simulink model "Problem3_sim"  (R2018a)
settings: Solver=ode45  StartTime=0.0  StopTime=sim_time  RelTol=1e-3
values from neighbouring files (symbols this model uses):
  g = 9.81    [Problem3.m]
  kd_fi = (2*zeta_fi*omega_fi-alpha_fi1)/alpha_fi2    [Problem3.m]
  ki_chi = omega_chi^2*V_g/g    [Problem3.m]
  ki_fi = -0    (= 0)    [Problem3.m]
  kp_chi = 2*zeta_chi*omega_chi*V_g/g    [Problem3.m]
  kp_fi = -2    [Problem3.m]
  sim_time = 600    [Problem3.m]
  V_g = 580/3.6    (= 161.111111111)    [Problem3.m]
undefined symbols (not defined in the file or in its folder): data
libraries: simulink_extras x2
settings Model: Creator=marti  LastModifiedBy=Anders Vagle
settings OptimizationCC: LifeSpan=inf
settings DebuggingCC: SFExecutionAtInitializationDiag=none
settings HardwareCC: ProdBitPerSizeT=32  ProdBitPerPtrDiffT=32  ProdWordSize=32  ProdHWDeviceType=Specified
settings CodeAppCC: StateflowObjectComments=on

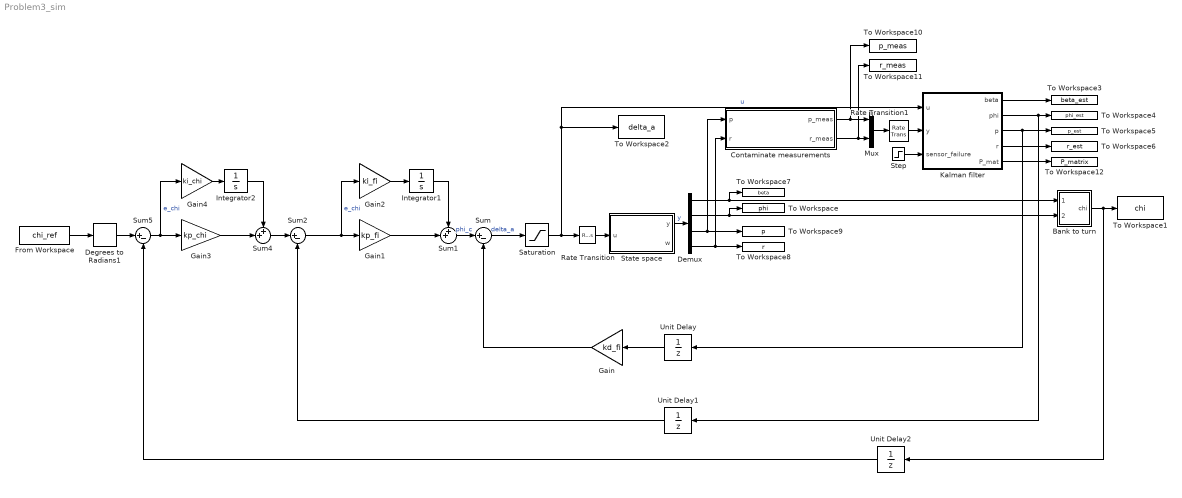
== system Problem3_sim ==
  Bank to turn : Subsystem
  Contaminate measurements : MATLAB Function  TreatAsAtomicUnit=on
  Degrees to Radians1 : simulink_extras/Transformations/Degrees to Radians
  Demux : Demux
  From Workspace : FromWorkspace  VariableName=chi_ref  SampleTime=0  Interpolate=off  OutputAfterFinalValue=Holding final value
  Gain : Gain  Gain=kd_fi
  Gain1 : Gain  Gain=kp_fi
  Gain2 : Gain  Gain=ki_fi
  Gain3 : Gain  Gain=kp_chi
  Gain4 : Gain  Gain=ki_chi
  Integrator1 : Integrator
  Integrator2 : Integrator
  Kalman filter : MATLAB Function  TreatAsAtomicUnit=on  mask{data=data}
      mask prompts: data "data struct"
  Mux : Mux  Inputs=2
  Rate Transition : RateTransition  OutPortSampleTime=Ts
  Rate Transition1 : RateTransition
  Saturation : Saturate  UpperLimit=30/180*pi  LowerLimit=-30/180*pi
  State space : MATLAB Function  TreatAsAtomicUnit=on
  Step : Step  Time=sim_time*2  SampleTime=0
  Sum : Sum  Inputs=|+-
  Sum1 : Sum  Inputs=++|
  Sum2 : Sum  Inputs=|+-
  Sum4 : Sum  Inputs=++|
  Sum5 : Sum  Inputs=|+-
  To Workspace : ToWorkspace  VariableName=phi  SaveFormat=Timeseries  SampleTime=-1
  To Workspace1 : ToWorkspace  VariableName=chi  SaveFormat=Timeseries  SampleTime=-1
  To Workspace10 : ToWorkspace  VariableName=p_meas  SaveFormat=Timeseries  SampleTime=-1
  To Workspace11 : ToWorkspace  VariableName=r_meas  SaveFormat=Timeseries  SampleTime=-1
  To Workspace12 : ToWorkspace  VariableName=P_matrix  SampleTime=-1
  To Workspace2 : ToWorkspace  VariableName=delta_a  SaveFormat=Timeseries  SampleTime=-1
  To Workspace3 : ToWorkspace  VariableName=beta_est  SaveFormat=Timeseries  SampleTime=-1
  To Workspace4 : ToWorkspace  VariableName=phi_est  SaveFormat=Timeseries  SampleTime=-1
  To Workspace5 : ToWorkspace  VariableName=p_est  SaveFormat=Timeseries  SampleTime=-1
  To Workspace6 : ToWorkspace  VariableName=r_est  SaveFormat=Timeseries  SampleTime=-1
  To Workspace7 : ToWorkspace  VariableName=beta  SaveFormat=Timeseries  SampleTime=-1
  To Workspace8 : ToWorkspace  VariableName=r  SaveFormat=Timeseries  SampleTime=-1
  To Workspace9 : ToWorkspace  VariableName=p  SaveFormat=Timeseries  SampleTime=-1
  Unit Delay : UnitDelay  SampleTime=-1
  Unit Delay1 : UnitDelay  SampleTime=-1
  Unit Delay2 : UnitDelay  SampleTime=-1
  wires:
  Gain/1 -> Sum/2
  Sum1/1 -> Sum/1  "phi_c"
  Integrator1/1 -> Sum1/1
  Gain1/1 -> Sum1/2
  Sum2/1 -> Gain2/1, Gain1/1  "e_chi"
  Demux/2 -> To Workspace/1, Bank to turn/2(phi)
  Integrator2/1 -> Sum4/1
  Gain3/1 -> Sum4/2
  Sum5/1 -> Gain4/1, Gain3/1  "e_chi"
  Sum/1 -> Saturation/1  "delta_a"
  Sum4/1 -> Sum2/1
  Degrees to Radians1/1 -> Sum5/1
  From Workspace/1 -> Degrees to Radians1/1
  Demux/1 -> To Workspace7/1, Bank to turn/1(beta)
  Saturation/1 -> Rate Transition/1, Kalman filter/1(u), To Workspace2/1  "u"
  State space/1(y) -> Demux/1  "y"
  Demux/3 -> To Workspace9/1, Contaminate measurements/1(p)
  Gain2/1 -> Integrator1/1
  Gain4/1 -> Integrator2/1
  Demux/4 -> Contaminate measurements/2(r), To Workspace8/1
  Contaminate measurements/2(r_meas) -> To Workspace11/1, Mux/2
  Contaminate measurements/1(p_meas) -> Mux/1, To Workspace10/1
  Kalman filter/1(beta) -> To Workspace3/1
  Kalman filter/2(phi) -> Unit Delay1/1, To Workspace4/1
  Kalman filter/3(p) -> Unit Delay/1, To Workspace5/1
  Kalman filter/4(r) -> To Workspace6/1
  Rate Transition/1 -> State space/1(u)
  Unit Delay/1 -> Gain/1
  Unit Delay1/1 -> Sum2/2
  Mux/1 -> Rate Transition1/1
  Rate Transition1/1 -> Kalman filter/2(y)
  Unit Delay2/1 -> Sum5/2
  Bank to turn/1(chi) -> To Workspace1/1, Unit Delay2/1
  Kalman filter/5(P_mat) -> To Workspace12/1
  Step/1 -> Kalman filter/3(sensor_failure)

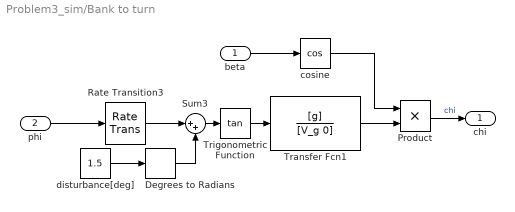
== system Problem3_sim/Bank to turn ==
  beta : Inport
  phi : Inport  Port=2
  Degrees to Radians : simulink_extras/Transformations/Degrees to Radians
  Product : Product
  Rate Transition3 : RateTransition  OutPortSampleTime=Ts
  Sum3 : Sum  Inputs=|++
  Transfer Fcn1 : TransferFcn  Numerator=[g]  Denominator=[V_g 0]
  Trigonometric Function : Trigonometry  Operator=tan
  cosine : Trigonometry  Operator=cos
  disturbance[deg] : Constant  Value=1.5
  chi : Outport
  wires:
  cosine/1 -> Product/1
  phi/1 -> Rate Transition3/1
  beta/1 -> cosine/1
  disturbance[deg]/1 -> Degrees to Radians/1
  Trigonometric Function/1 -> Transfer Fcn1/1
  Rate Transition3/1 -> Sum3/1
  Sum3/1 -> Trigonometric Function/1
  Degrees to Radians/1 -> Sum3/2
  Transfer Fcn1/1 -> Product/2
  Product/1 -> chi/1  "chi"

== matlab function Problem3_sim/Contaminate measurements ==
  data: p input; p_meas output; r input; r_meas output
function [p_meas, r_meas] = contaminate(p, r)

% persistent counter; % Variable for checking if it is the first iteration.
% coder.extrinsic('randn','rng');
% if isempty(counter)
%    counter = 1;
%    rng('shuffle'); % Necessary for generating unique process noise for every simulation.
% end

% var_p = 0.2^2;
% var_r = 0.2^2;

p_meas = p + randn(1,1)*sqrt((0.2*pi/180)^2);
r_meas = r + randn(1,1)*sqrt((0.2*pi/180)^2);

== matlab function Problem3_sim/State space ==
  data: u input; y output; w output
function [y, w] = state_space(u)
% Generate the output of the state space

    % Persistent variables to be kept between function calls
    persistent counter; % Variable for checking if it is the first iteration.
    persistent x;       % The state x
    
   % The next line is necessary for generating unique process noise for every simulation.
   % Otherwise, the noise will be equal every time you run the simulation,
   % even though it is white. This has to do with how Matlab generates
   % random numbers. 
   %coder.extrinsic('randn','rng');
    
    h = 0.01;       % Time step of Euler integration
    delta_a_c = u;  % Aileron input
    
    if isempty(counter)
      % First iteration
        counter = 1;
           
        % Initialize state space
        x = zeros(5,1);
        w = zeros(5,1); 
        rng(100); % Necessary for generating unique process noise for every simulation.
    
    else
        % State-space matrices
        A = [-0.322, 0.052, 0.028, -1.12, 0.002;
             0, 0, 1, -0.001, 0;
             -10.6, 0, -2.87, 0.46, -0.65;
             6.87, 0, -0.04, -0.32, -0.02;
             0, 0, 0, 0, -7.5];
 
        B = [0; 0; 0; 0; 7.5;];
        
        E = eye(5);
        
        % Discrete version
        Ad = eye(5) + h*A;
        Bd = h*B;
        Ed = E;
        
        % The Qd matrix in the assignment is given directly in discrete-time here and
        % therefore, it is not necessary to discretize E.
        Qd = h*10^-6*[0.001, 0, 0, 0, 0;
                  0, 1, 0, 0, 0;
                  0, 0, 100, 0, 0;
                  0, 0, 0, 10, 0;
                  0, 0, 0, 0, 0];
          
        w = sqrt(Qd)*randn(5,1,1); % The standard deviation must be multiplied with random numbers with a zero-mean unit variance random number to generate process noise. 
        
        % Discrete-time state space update
        x = Ad*x + Bd * delta_a_c + Ed*w;
    end
    y = x(1:4); % Return every state except the actuator state.
end

== matlab function Problem3_sim/Kalman filter ==
  settings: updateMethod=DISCRETE  sampleTime=Ts
  data: beta output; u input; y input; sensor_failure input; data parameter; phi output; p output; r output; P_mat output
function [beta,phi,p,r, P_mat]  = Kalman_filter(u,y,sensor_failure,data)
persistent xpri xhat P;

A = data.A;
B = data.B;
C = data.C;
Q = data.Q;
R = data.R;
I = data.I;
E = data.E;

if isempty(xpri)
    xpri = data.xhat0;
    P = data.P;
end

if sensor_failure
    R = [1000000 0; 0 1000000];
end

K = P*C'/(C*P*C' + R);
xhat = xpri + K*(y - C*xpri);
P = (I - K*C)*P*(I - K*C)' + K*R*K';

xpri = A*xhat + B*u;
P = A*P*A' + E*Q*E';
P_mat = P;

beta = xhat(1);
phi = xhat(2);
p = xhat(3);
r = xhat(4);
